simulink model "BLDC2017a"  (R2024a)
settings: Solver=VariableStepAuto  StartTime=0.0  StopTime=10.0  RelTol=1e-3
model workspace (MAT data in the model file):
  NULL = 1
libraries: slrealtimeiplib x2, spsControlledVoltageSourceLib x1, spsPermanentMagnetSynchronousMachineLib x1, spsUniversalBridgeLib x1
settings Model: Creator=d  LastModifiedBy=d
settings SolverCC: AlgebraicLoopSolver=TrustRegion
settings DebuggingCC: ArithmeticOperatorsInVariantConditions=warning
settings SFSimCC: CustomCodeUndefinedFunction=UseInterfaceOnly
settings RTWCC: GPUComputeCapability=3.5
settings CodeAppCC: StateflowObjectComments=on

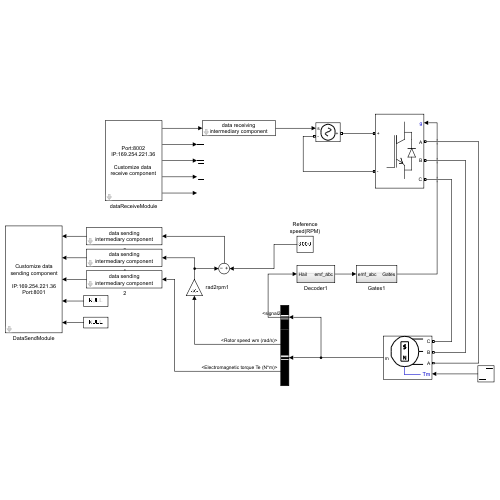
[thumbnail: Simulink's stored preview of the top-level diagram]
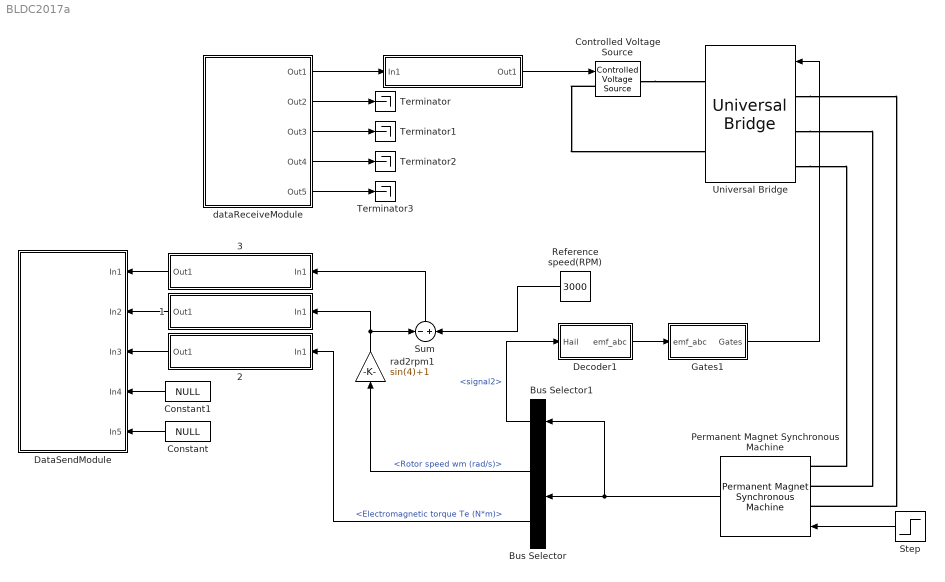
== system BLDC2017a ==
  " " : Subsystem
      mask DialogControl ParameterGroupVar Prompt: 参数
      mask Display: disp('data receiving\nintermediary component');
  " 1" : Subsystem
      mask DialogControl ParameterGroupVar Prompt: 参数
      mask Display: disp('data sending\nintermediary component');
  " 2" : Subsystem
      mask DialogControl ParameterGroupVar Prompt: 参数
      mask Display: disp('data sending\nintermediary component');
  " 3" : Subsystem
      mask DialogControl ParameterGroupVar Prompt: 参数
      mask Display: disp('data sending\nintermediary component');
  Bus Selector : BusSelector  OutputSignals=Rotor speed wm (rad/s),Electromagnetic torque Te (N*m)
  Bus Selector1 : BusSelector  OutputSignals=signal2
  Constant : Constant  Value=NULL
  Constant1 : Constant  Value=NULL
  Controlled Voltage Source : spsControlledVoltageSourceLib/Controlled Voltage Source  Initialize=on  Source_Type=AC  Amplitude=0  Phase=0  Frequency=0  Measurements=None
  DataSendModule : Subsystem
      mask DialogControl ParameterGroupVar Prompt: 参数
      mask Display: disp('Customize data\nsending component\n\nIP:169.254.221.36\nPort:8001');
  Decoder1 : Subsystem
  Gates1 : Subsystem
  Permanent Magnet Synchronous Machine : spsPermanentMagnetSynchronousMachineLib/Permanent Magnet Synchronous Machine  NbPhases=3  FluxDistribution=Sinusoidal  RotorType=Round  MechanicalLoad=Torque Tm  PresetModel=No  ShowDetailedParameters=on  MeasurementBus=off  Resistance=0.0485  Inductance=8.5e-3  dqInductances=[8.5e-3,8.5e-3]  La=0.000395  MachineConstant=Flux linkage established by magnets (V.s)  Flux=0.1194  VoltageCst=86.6271  TorqueCst=0.7164  Flat=120  Mechanical=[0.0027 0.0004924 4 0]  PolePairs=4  InitialConditions=[0,0, 0,0]  InitialConditions5ph=[0 0 0 0 0 0]  RefAngle=90 degrees behind phase A axis (modified Park)  IterativeDiscreteModel=Trapezoidal non iterative  TsBlock=-1  TsPowergui=0
  Reference speed(RPM) : Constant  Value=3000
  Step : Step  SampleTime=0
  Sum : Sum  Inputs=-|+
  Terminator{,1..3} (4 alike) : Terminator
  Universal Bridge : spsUniversalBridgeLib/Universal Bridge  Arms=3  SnubberResistance=1e5  SnubberCapacitance=inf  Device=IGBT / Diodes  Ron=1e-3  Lon=0  ForwardVoltages="[  0  0  ]"  ForwardVoltage=0  GTOparameters=[ 10e-6 , 20e-6 ]  IGBTparameters=[ 1e-6 , 2e-6 ]  Measurements=None  Measurements_2=None  converterType=Rectifier
  dataReceiveModule : Subsystem
      mask DialogControl ParameterGroupVar Prompt: 参数
      mask Display: disp('Port:8002\nIP:169.254.221.36\n\nCustomize data \nreceive component');
  rad2rpm1 : Gain  Gain=sin(4)+1
  wires:
  dataReceiveModule/2(Out2) -> Terminator/1
  dataReceiveModule/4(Out4) -> Terminator2/1
  dataReceiveModule/3(Out3) -> Terminator1/1
  dataReceiveModule/5(Out5) -> Terminator3/1
  dataReceiveModule/1(Out1) -> " "/1(In1)
  " "/1(Out1) -> Controlled Voltage Source/1
  Step/1 -> Permanent Magnet Synchronous Machine/1
  Permanent Magnet Synchronous Machine/1 -> Bus Selector1/1, Bus Selector/1
  Bus Selector/1 -> rad2rpm1/1  "<Rotor speed wm (rad/s)>"
  Bus Selector1/1 -> Decoder1/1(Hail)  "<signal2>"
  Decoder1/1(emf_abc) -> Gates1/1(emf_abc)
  Gates1/1(Gates) -> Universal Bridge/1
  Constant/1 -> DataSendModule/5(In5)
  Constant1/1 -> DataSendModule/4(In4)
  " 2"/1(Out1) -> DataSendModule/3(In3)
  " 3"/1(Out1) -> DataSendModule/1(In1)
  Reference speed(RPM)/1 -> Sum/2
  rad2rpm1/1 -> " 1"/1(In1), Sum/1
  Sum/1 -> " 3"/1(In1)
  " 1"/1(Out1) -> DataSendModule/2(In2)
  Bus Selector/2 -> " 2"/1(In1)  "<Electromagnetic torque Te (N*m)>"
  connections:
  Controlled Voltage Source/RConn1 -- Universal Bridge/RConn1
  Controlled Voltage Source/LConn1 -- Universal Bridge/RConn2
  Universal Bridge/LConn1 -- Permanent Magnet Synchronous Machine/LConn1
  Universal Bridge/LConn2 -- Permanent Magnet Synchronous Machine/LConn2
  Universal Bridge/LConn3 -- Permanent Magnet Synchronous Machine/LConn3

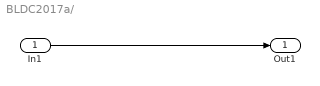
== system BLDC2017a/  ==
  In1 : Inport
  Out1 : Outport
  wires:
  In1/1 -> Out1/1

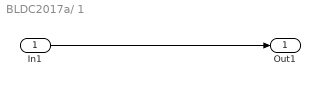
== system BLDC2017a/ 1 ==
  In1 : Inport
  Out1 : Outport
  wires:
  In1/1 -> Out1/1

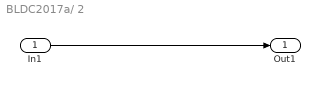
== system BLDC2017a/ 2 ==
  In1 : Inport
  Out1 : Outport
  wires:
  In1/1 -> Out1/1

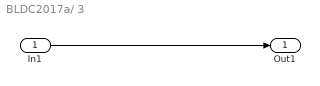
== system BLDC2017a/ 3 ==
  In1 : Inport
  Out1 : Outport
  wires:
  In1/1 -> Out1/1

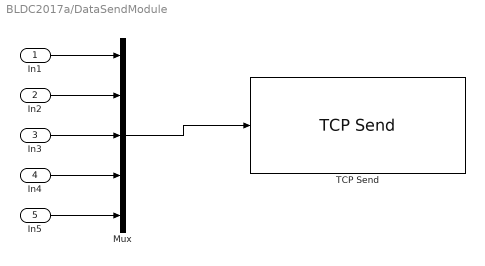
== system BLDC2017a/DataSendModule ==
  In1 : Inport
  In2 : Inport  Port=2
  In3 : Inport  Port=3
  In4 : Inport  Port=4
  In5 : Inport  Port=5
  Mux : Mux  Inputs=5
  TCP Send : slrealtimeiplib/TCP Send  socketAddPortVal=<empty>  sampleTime=-1
  wires:
  In1/1 -> Mux/1
  In2/1 -> Mux/2
  In3/1 -> Mux/3
  In4/1 -> Mux/4
  In5/1 -> Mux/5
  Mux/1 -> TCP Send/2

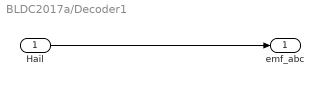
== system BLDC2017a/Decoder1 ==
  Hail : Inport
  emf_abc : Outport
  wires:
  Hail/1 -> emf_abc/1

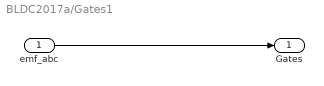
== system BLDC2017a/Gates1 ==
  emf_abc : Inport
  Gates : Outport
  wires:
  emf_abc/1 -> Gates/1

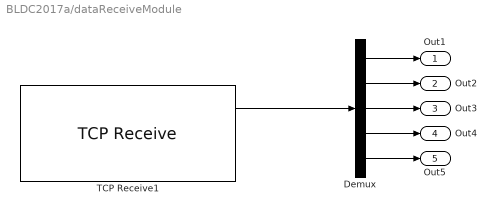
== system BLDC2017a/dataReceiveModule ==
  Demux : Demux  Outputs=5
  TCP Receive1 : slrealtimeiplib/TCP Receive  socketAddPortVal=<empty>  rcvWidth=16  sampleTime=-1
  Out1 : Outport
  Out2 : Outport  Port=2
  Out3 : Outport  Port=3
  Out4 : Outport  Port=4
  Out5 : Outport  Port=5
  wires:
  Demux/1 -> Out1/1
  Demux/2 -> Out2/1
  Demux/3 -> Out3/1
  Demux/4 -> Out4/1
  Demux/5 -> Out5/1
  TCP Receive1/1 -> Demux/1
